simulink model "SIMULATION_MODEL"  (R2024b)
settings: Solver=VariableStepAuto  StartTime=0.0  StopTime=inf  MaxStep=0.2  RelTol=1e-3
undefined symbols (not defined in the file or in its folder): juliandate, R, sat
libraries: matrix_library x4, aerolibutil x4, sharedtransform x2, sharedutil x1, simulink_extras x1
settings Model: Creator=Ameya  LastModifiedBy=Ameya

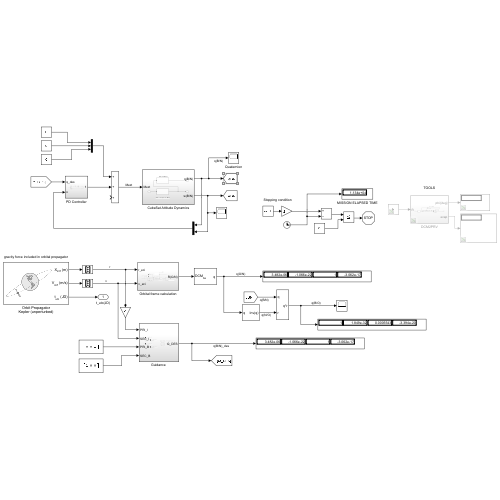
[thumbnail: Simulink's stored preview of the top-level diagram]
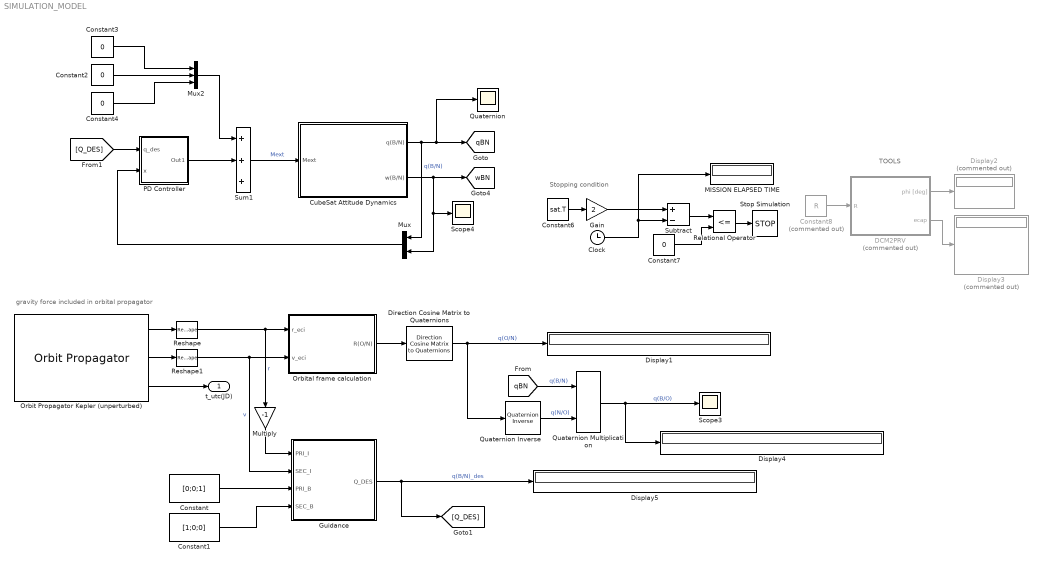
== system SIMULATION_MODEL ==
  note: TOOLS
  note: Stopping condition
  note: gravity force included in orbital propagator
  Clock : Clock
  Constant : Constant  Value=[0;0;1]  SampleTime=-1
  Constant1 : Constant  Value=[1;0;0]  SampleTime=-1
  Constant{2..4,7} (4 alike) : Constant  Value=0
  Constant6 : Constant  Value=sat.T
  Constant8 : Constant  Commented=on  Value=R
  CubeSat Attitude Dynamics : Subsystem
  DCM2PRV : Subsystem  Commented=on
  Direction Cosine Matrix to Quaternions : sharedtransform/Direction Cosine Matrix  to Quaternions  aMode=0  action=Error  tolerance=eps(2)
      settings: LibrarySourceBlock=|
      | aerolibtransform2/Direction Cosine Matrix
      | to Quaternions
  Display1 : Display
  Display2 : Display  Commented=on
  Display3 : Display  Commented=on
  Display4 : Display
  Display5 : Display
  Gain : Gain  Gain=2
  "Guidance " : Subsystem
  MISSION ELAPSED TIME : Display
  Multiply : Gain  Gain=-1
  Mux : Mux  Inputs=2
  Mux2 : Mux  Inputs=3
  Orbit Propagator Kepler (unperturbed) : OrbitPropagator  accelIn=on  startDate=juliandate(2025, 1, 1, 6, 0, 0)  semiMajorAxis=sat.a  eccentricity=sat.e  inclination=rad2deg(sat.i)  raan=rad2deg(sat.RAAN)  argPeriapsis=rad2deg(sat.w)  trueAnomaly=rad2deg(sat.ta)  inertialPosition=[3649700.0 3308200.0 -4676600.0]  inertialVelocity=[-2750.8 6666.4 2573.4]  fixedPosition=[-4142689.0 -2676864.7 -4669861.6]  fixedVelocity=[1452.7 -6720.7 2568.1]  gravityModel=Oblate ellipsoid (J2)  customR=3396200  customMu=4.305e13  customJ2=1.0826269e-03  customOmega=4.06125949e-3
  Orbital frame calculation : Subsystem
  PD Controller : Subsystem
  Quaternion : Scope
  Quaternion Inverse : aerolibutil/Quaternion Inverse
  Quaternion Multiplication : aerolibutil/Quaternion Multiplication
  Relational Operator : RelationalOperator  Operator=<=  OutDataTypeStr=boolean  RndMeth=Simplest  InputSameDT=off
  Reshape : Reshape  OutputDimensionality=Column vector (2-D)
  Reshape1 : Reshape  OutputDimensionality=Column vector (2-D)
  Scope3 : Scope
  Scope4 : Scope
  Stop Simulation : Stop
  Subtract : Sum  Inputs=+-
  Sum1 : Sum  Inputs=+++
  t_utc(JD) : Outport
  tag scope: qBN=global, wBN=global
  wires:
  Clock/1 -> MISSION ELAPSED TIME/1, Subtract/2
  Constant4/1 -> Mux2/3
  Constant7/1 -> Relational Operator/2
  Relational Operator/1 -> Stop Simulation/1
  DCM2PRV/1(phi [deg]) -> Display2/1
  Constant3/1 -> Mux2/1
  Subtract/1 -> Relational Operator/1
  Mux2/1 -> Sum1/1
  DCM2PRV/2(ecap) -> Display3/1
  Constant6/1 -> Gain/1
  CubeSat Attitude Dynamics/1(q(B/N)) -> Mux/1, [qBN], Quaternion/1  "q(B/N)"
  Sum1/1 -> CubeSat Attitude Dynamics/1(Mext)  "Mext"
  CubeSat Attitude Dynamics/2(w(B/N)) -> Mux/2, Scope4/1, [wBN]
  Constant8/1 -> DCM2PRV/1(R)
  Gain/1 -> Subtract/1
  Constant2/1 -> Mux2/2
  Orbital frame calculation/1(R(O/N)) -> Direction Cosine Matrix to Quaternions/1
  Quaternion Multiplication/1 -> Display4/1, Scope3/1  "q(B/O)"
  Orbit Propagator Kepler (unperturbed)/1 -> Reshape/1
  Orbit Propagator Kepler (unperturbed)/3 -> t_utc(JD)/1
  [qBN] -> Quaternion Multiplication/1  "q(B/N)"
  Reshape/1 -> Multiply/1, Orbital frame calculation/1(r_eci)  "r"
  Reshape1/1 -> Orbital frame calculation/2(v_eci), "Guidance "/2(SEC_I)  "v"
  Quaternion Inverse/1 -> Quaternion Multiplication/2  "q(N/O)"
  Direction Cosine Matrix to Quaternions/1 -> Display1/1, Quaternion Inverse/1  "q(O/N)"
  Orbit Propagator Kepler (unperturbed)/2 -> Reshape1/1
  "Guidance "/1(Q_DES) -> [Q_DES], Display5/1  "q(B/N)_des"
  Constant/1 -> "Guidance "/3(PRI_B)
  Constant1/1 -> "Guidance "/4(SEC_B)
  Multiply/1 -> "Guidance "/1(PRI_I)
  [Q_DES] -> PD Controller/1(q_des)
  PD Controller/1(Out1) -> Sum1/2
  Mux/1 -> PD Controller/2(x)

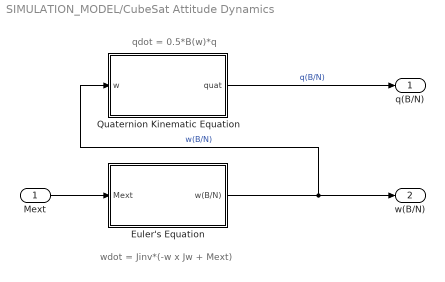
== system SIMULATION_MODEL/CubeSat Attitude Dynamics ==
  note: qdot = 0.5*B(w)*q
  note: wdot = Jinv*(-w x Jw + Mext)
  Mext : Inport
  Euler's Equation : Subsystem
  Quaternion Kinematic Equation : Subsystem
  q(B/N) : Outport
  w(B/N) : Outport  Port=2
  wires:
  Mext/1 -> Euler's Equation/1(Mext)
  Euler's Equation/1(w(B/N)) -> Quaternion Kinematic Equation/1(w), w(B/N)/1  "w(B/N)"
  Quaternion Kinematic Equation/1(quat) -> q(B/N)/1  "q(B/N)"

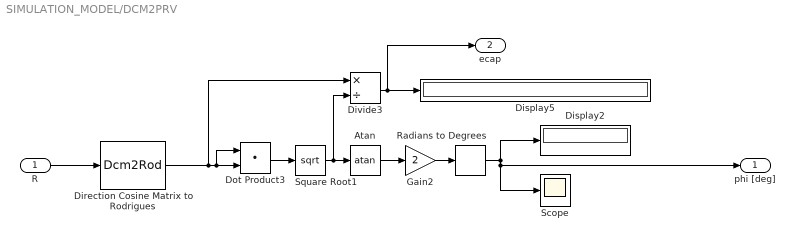
== system SIMULATION_MODEL/DCM2PRV ==
  R : Inport
  Atan : Trigonometry  Operator=atan
  Direction Cosine Matrix to Rodrigues : Dcm2Rod
  Display2 : Display
  Display5 : Display
  Divide3 : Product  Inputs=*/
  Dot Product3 : DotProduct  OutDataTypeStr=Inherit: Inherit via internal rule
  Gain2 : Gain  Gain=2
  Radians to Degrees : simulink_extras/Transformations/Radians to Degrees
  Scope : Scope
  Square Root1 : Sqrt
  phi [deg] : Outport
  ecap : Outport  Port=2
  wires:
  Radians to Degrees/1 -> phi [deg]/1, Scope/1, Display2/1
  Divide3/1 -> ecap/1, Display5/1
  R/1 -> Direction Cosine Matrix to Rodrigues/1
  Square Root1/1 -> Divide3/2, Atan/1
  Atan/1 -> Gain2/1
  Direction Cosine Matrix to Rodrigues/1 -> Divide3/1, Dot Product3/2, Dot Product3/1
  Dot Product3/1 -> Square Root1/1
  Gain2/1 -> Radians to Degrees/1

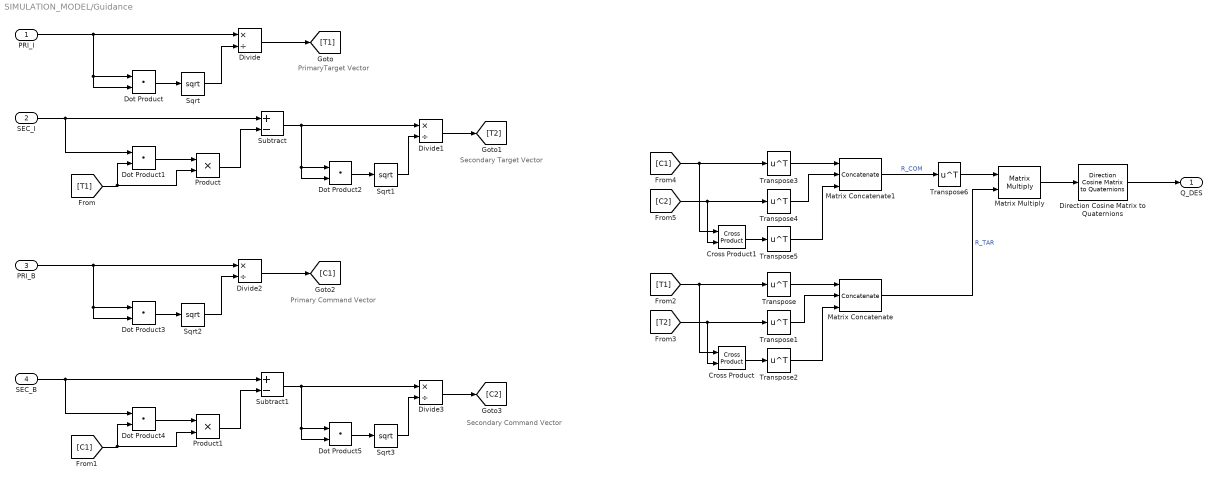
== system SIMULATION_MODEL/Guidance  ==
  note: PrimaryTarget Vector
  note: Secondary Target Vector
  note: Primary Command Vector
  note: Secondary Command Vector
  PRI_I : Inport
  SEC_I : Inport  Port=2
  PRI_B : Inport  Port=3
  SEC_B : Inport  Port=4
  Cross Product : matrix_library/Cross Product
  Cross Product1 : matrix_library/Cross Product
  Direction Cosine Matrix to Quaternions : sharedtransform/Direction Cosine Matrix  to Quaternions  aMode=0  action=None  tolerance=eps(2)
      settings: LibrarySourceBlock=|
      | aerolibtransform2/Direction Cosine Matrix
      | to Quaternions
  Divide{,1..3} (4 alike) : Product  Inputs=*/
  Dot Product{,1..5} (6 alike) : DotProduct  OutDataTypeStr=Inherit: Inherit via internal rule
  Matrix Concatenate : Concatenate  NumInputs=3  Mode=Multidimensional array
  Matrix Concatenate1 : Concatenate  NumInputs=3  Mode=Multidimensional array
  Matrix Multiply : Product  Multiplication=Matrix(*)
  Product : Product
  Product1 : Product
  Sqrt{,1..3} (4 alike) : Sqrt
  Subtract : Sum  Inputs=+-
  Subtract1 : Sum  Inputs=+-
  Transpose{,1..6} (7 alike) : Math  Operator=transpose
  Q_DES : Outport
  wires:
  PRI_I/1 -> Dot Product/2, Dot Product/1, Divide/1
  Dot Product/1 -> Sqrt/1
  Divide/1 -> [T1]
  Transpose/1 -> Matrix Concatenate/1
  SEC_I/1 -> Subtract/1, Dot Product1/1
  Sqrt/1 -> Divide/2
  Dot Product1/1 -> Product/1
  [T1] -> Product/2, Dot Product1/2
  Product/1 -> Subtract/2
  Sqrt1/1 -> Divide1/2
  Dot Product2/1 -> Sqrt1/1
  Subtract/1 -> Divide1/1, Dot Product2/2, Dot Product2/1
  Divide1/1 -> [T2]
  Sqrt2/1 -> Divide2/2
  Dot Product3/1 -> Sqrt2/1
  PRI_B/1 -> Dot Product3/2, Dot Product3/1, Divide2/1
  Divide2/1 -> [C1]
  Dot Product5/1 -> Sqrt3/1
  Sqrt3/1 -> Divide3/2
  Product1/1 -> Subtract1/2
  Divide3/1 -> [C2]
  [C1] -> Product1/2, Dot Product4/2
  Subtract1/1 -> Divide3/1, Dot Product5/2, Dot Product5/1
  Dot Product4/1 -> Product1/1
  SEC_B/1 -> Subtract1/1, Dot Product4/1
  Transpose1/1 -> Matrix Concatenate/2
  Transpose2/1 -> Matrix Concatenate/3
  [T1] -> Cross Product/1, Transpose/1
  [T2] -> Cross Product/2, Transpose1/1
  Cross Product/1 -> Transpose2/1
  Matrix Concatenate/1 -> Matrix Multiply/2  "R_TAR"
  Cross Product1/1 -> Transpose5/1
  [C1] -> Cross Product1/1, Transpose3/1
  Transpose3/1 -> Matrix Concatenate1/1
  Transpose4/1 -> Matrix Concatenate1/2
  Transpose5/1 -> Matrix Concatenate1/3
  [C2] -> Cross Product1/2, Transpose4/1
  Matrix Concatenate1/1 -> Transpose6/1  "R_COM"
  Transpose6/1 -> Matrix Multiply/1
  Matrix Multiply/1 -> Direction Cosine Matrix to Quaternions/1
  Direction Cosine Matrix to Quaternions/1 -> Q_DES/1

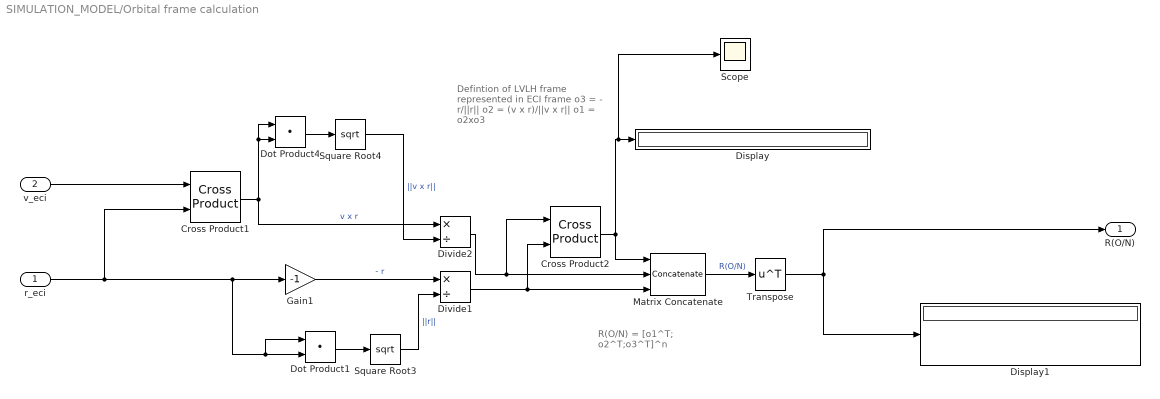
== system SIMULATION_MODEL/Orbital frame calculation ==
  note: R(O/N) = [o1^T; o2^T;o3^T]^n
  note: Defintion of LVLH frame
      | represented in ECI frame
      | o3 = - r/||r||
      | o2 = (v x r)/||v x r||
      | o1 = o2xo3
  r_eci : Inport
  v_eci : Inport  Port=2
  Cross Product1 : matrix_library/Cross Product
  Cross Product2 : matrix_library/Cross Product
  Display : Display
  Display1 : Display
  Divide1 : Product  Inputs=*/
  Divide2 : Product  Inputs=*/
  Dot Product1 : DotProduct  OutDataTypeStr=Inherit: Inherit via internal rule
  Dot Product4 : DotProduct  OutDataTypeStr=Inherit: Inherit via internal rule
  Gain1 : Gain  Gain=-1
  Matrix Concatenate : Concatenate  NumInputs=3  Mode=Multidimensional array  ConcatenateDimension=2
  Scope : Scope
  Square Root3 : Sqrt
  Square Root4 : Sqrt
  Transpose : Math  Operator=transpose
  R(O/N) : Outport
  wires:
  Cross Product2/1 -> Scope/1, Display/1, Matrix Concatenate/1
  Divide2/1 -> Cross Product2/1, Matrix Concatenate/2
  Cross Product1/1 -> Dot Product4/2, Dot Product4/1, Divide2/1  "v x r"
  r_eci/1 -> Cross Product1/2, Dot Product1/1, Dot Product1/2, Gain1/1
  Gain1/1 -> Divide1/1  "- r"
  Square Root3/1 -> Divide1/2  "||r||"
  Square Root4/1 -> Divide2/2  "||v x r||"
  Dot Product1/1 -> Square Root3/1
  v_eci/1 -> Cross Product1/1
  Matrix Concatenate/1 -> Transpose/1  "R(O/N)"
  Divide1/1 -> Cross Product2/2, Matrix Concatenate/3
  Dot Product4/1 -> Square Root4/1
  Transpose/1 -> Display1/1, R(O/N)/1

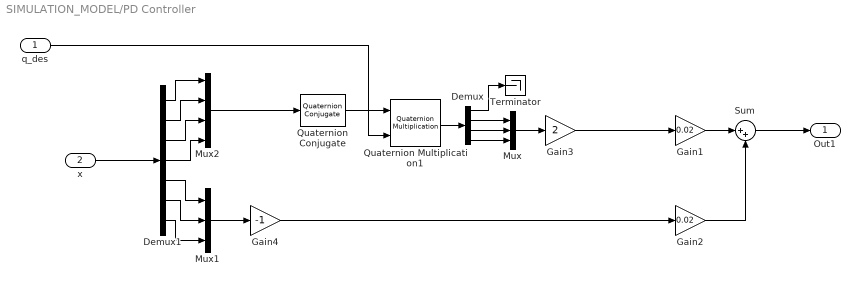
== system SIMULATION_MODEL/PD Controller ==
  q_des : Inport
  x : Inport  Port=2
  Demux : Demux
  Demux1 : Demux  Outputs=7
  Gain1 : Gain  Gain=0.02
  Gain2 : Gain  Gain=0.02
  Gain3 : Gain  Gain=2
  Gain4 : Gain  Gain=-1
  Mux : Mux  Inputs=3
  Mux1 : Mux  Inputs=3
  Mux2 : Mux
  Quaternion Conjugate : aerolibutil/Quaternion Conjugate
  Quaternion Multiplication1 : aerolibutil/Quaternion Multiplication
  Sum : Sum  Inputs=|++
  Terminator : Terminator
  Out1 : Outport
  wires:
  Demux/2 -> Mux/1
  Demux/4 -> Mux/3
  Gain3/1 -> Gain1/1
  Demux/3 -> Mux/2
  Gain2/1 -> Sum/2
  Quaternion Multiplication1/1 -> Demux/1
  Gain4/1 -> Gain2/1
  x/1 -> Demux1/1
  Quaternion Conjugate/1 -> Quaternion Multiplication1/1
  Gain1/1 -> Sum/1
  Mux/1 -> Gain3/1
  Demux/1 -> Terminator/1
  Sum/1 -> Out1/1
  q_des/1 -> Quaternion Multiplication1/2
  Demux1/5 -> Mux1/1
  Demux1/6 -> Mux1/2
  Demux1/7 -> Mux1/3
  Mux1/1 -> Gain4/1
  Demux1/4 -> Mux2/4
  Demux1/1 -> Mux2/1
  Demux1/2 -> Mux2/2
  Demux1/3 -> Mux2/3
  Mux2/1 -> Quaternion Conjugate/1

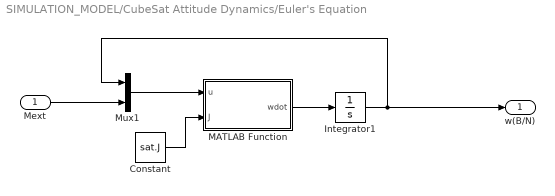
== system SIMULATION_MODEL/CubeSat Attitude Dynamics/Euler's Equation ==
  Mext : Inport
  Constant : Constant  Value=sat.J
  Integrator1 : Integrator  InitialCondition=sat.omegaBO
  MATLAB Function : MATLAB Function  TreatAsAtomicUnit=on
  Mux1 : Mux  Inputs=2
  w(B/N) : Outport
  wires:
  Mext/1 -> Mux1/2
  MATLAB Function/1(wdot) -> Integrator1/1
  Integrator1/1 -> Mux1/1, w(B/N)/1
  Mux1/1 -> MATLAB Function/1(u)
  Constant/1 -> MATLAB Function/2(J)

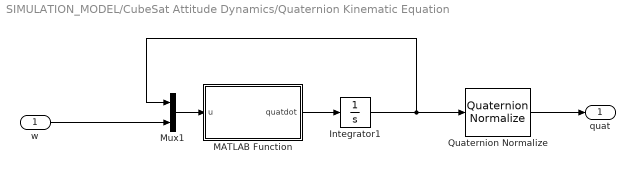
== system SIMULATION_MODEL/CubeSat Attitude Dynamics/Quaternion Kinematic Equation ==
  w : Inport
  Integrator1 : Integrator  InitialCondition=sat.quat
  MATLAB Function : MATLAB Function  TreatAsAtomicUnit=on
  Mux1 : Mux  Inputs=2
  Quaternion Normalize : sharedutil/Quaternion Normalize  aMode=aMode
  quat : Outport
  wires:
  Mux1/1 -> MATLAB Function/1(u)
  Integrator1/1 -> Quaternion Normalize/1, Mux1/1
  MATLAB Function/1(quatdot) -> Integrator1/1
  w/1 -> Mux1/2
  Quaternion Normalize/1 -> quat/1

== matlab function SIMULATION_MODEL/CubeSat Attitude Dynamics/Euler's Equation/MATLAB Function ==
  data: u input; wdot output; J input
function wdot = EulersEOM(u,J)
    w = u(1:3);
    m = u(4:6);
    wdot = J\(-cross(w,(J*w))+m);
end

== matlab function SIMULATION_MODEL/CubeSat Attitude Dynamics/Quaternion Kinematic Equation/MATLAB Function ==
  data: u input; quatdot output
function quatdot = quatKinematics(u)
    quat = u(1:4);
    p = u(5);
    q = u(6);
    r = u(7);
    quatdot = 0.5*[0,-p,-q,-r;
                p,0,r,-q;
                q,-r,0,p;
                r,q,-p,0]*quat;
end
